simulink model "golfmodel"  (R2015a)
settings: Solver=ode45  StartTime=0.0  StopTime=15  FixedStep=0.1  MaxStep=0.3  RelTol=1e-3
InitFcn:
  | K = 0.001;   % Constant for calculating drag
  | m = 0.045;   % Mass of a golf ball
  | vwind = 4.5; % Wind speed
values from neighbouring files (symbols this model uses):
  theta0 = angles(iOuter)    [golfmat.m]    (also in golfmatInner.m; golfmatOuter1.m; hit30deg.m = 0.523598775598; hit30degSol.m = 0.523598775598)
  v0 = velocities(iInner)    [golfmat.m]    (also in golfmatInner.m; golfmatOuter1.m; golfmatOuter2.m; golfsim.m = velocities(J))
settings Model: Creator=jrivitus  LastModifiedBy=hbrunnho
settings DataIOCC: SignalLoggingSaveFormat=ModelDataLogs  OutputTimes=0:0.1:10
settings OptimizationCC: ExpressionDepthLimit=2147483647  InitFltsAndDblsToZero=on
settings DebuggingCC: SaveWithParameterizedLinksMsg=none  UnderspecifiedInitializationDetection=Classic  MergeDetectMultiDrivingBlocksExec=none  SignalResolutionControl=TryResolveAllWithWarning  SolverPrmCheckMsg=warning  FcnCallInpInsideContextMsg=UseLocalSettings  StateNameClashWarn=warning
settings GRTTargetCC: TargetFcnLib=ansi_tfl_tmw.mat  CombineOutputUpdateFcns=off  GRTInterface=on

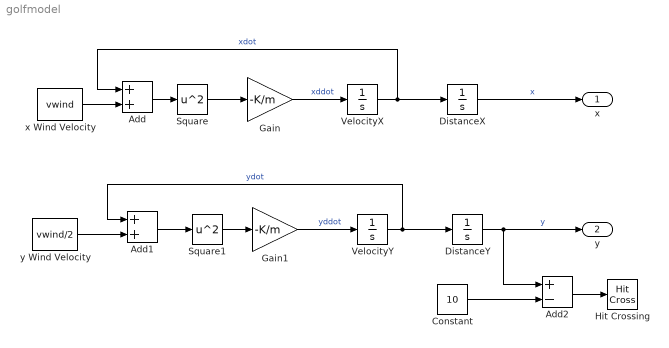
== system golfmodel ==
  Add : Sum
  Add1 : Sum
  Add2 : Sum  Inputs=+-
  Constant : Constant  Value=10
  DistanceX : Integrator
  DistanceY : Integrator
  Gain : Gain  Gain=-K/m
  Gain1 : Gain  Gain=-K/m
  Hit Crossing : HitCross  ShowOutputPort=off
  Square : Math  Operator=square  SaturateOnIntegerOverflow=on
  Square1 : Math  Operator=square  SaturateOnIntegerOverflow=on
  VelocityX : Integrator  InitialCondition=v0*cos(theta0)
  VelocityY : Integrator  InitialCondition=v0*sin(theta0)
  x Wind Velocity : Constant  Value=vwind
  y Wind Velocity : Constant  Value=vwind/2
  x : Outport
  y : Outport  Port=2
  wires:
  VelocityY/1 -> DistanceY/1, Add1/1  "ydot"
  DistanceY/1 -> Add2/1, y/1  "y"
  DistanceX/1 -> x/1  "x"
  VelocityX/1 -> DistanceX/1, Add/1  "xdot"
  Gain/1 -> VelocityX/1  "xddot"
  x Wind Velocity/1 -> Add/2
  Add/1 -> Square/1
  Square/1 -> Gain/1
  Add1/1 -> Square1/1
  Square1/1 -> Gain1/1
  Gain1/1 -> VelocityY/1  "yddot"
  y Wind Velocity/1 -> Add1/2
  Add2/1 -> Hit Crossing/1
  Constant/1 -> Add2/2
